simulink model "sunVector_test"  (R2018b)
settings: Solver=VariableStepAuto  StartTime=0.0  StopTime=600  RelTol=1e-3
values from neighbouring files (symbols this model uses):
  utc_test = 137803367    [solarPressure_fullOrbit_test_init.m]    (also in solarPressure_test2_init.m; solarPressure_test_init.m; sunVector_test_init.m = 197208000)
libraries: sunVector_lib x1, time_Lib x1
settings Model: Creator=devantormey  LastModifiedBy=devantormey

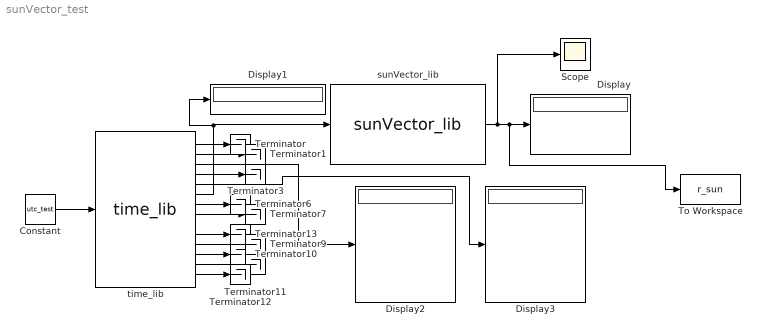
== system sunVector_test ==
  Constant : Constant  Value=utc_test
  Display{,1..3} (4 alike) : Display
  Scope : Scope
  Terminator{,1,3,6..7,9..13} (10 alike) : Terminator
  To Workspace : ToWorkspace  VariableName=r_sun  SaveFormat=Timeseries  SampleTime=-1
  sunVector_lib : sunVector_lib/sunVector_lib  SystemSampleTime=-1
  "time_lib " : time_Lib/time_lib    SystemSampleTime=-1
  wires:
  "time_lib "/3 -> Display2/1
  "time_lib "/12 -> Terminator10/1
  "time_lib "/2 -> Terminator1/1
  "time_lib "/4 -> Terminator3/1
  "time_lib "/13 -> Terminator11/1
  "time_lib "/11 -> Terminator9/1
  "time_lib "/7 -> Terminator6/1
  "time_lib "/8 -> Terminator7/1
  "time_lib "/1 -> Terminator/1
  "time_lib "/14 -> Terminator12/1
  "time_lib "/10 -> Terminator13/1
  Constant/1 -> "time_lib "/1
  "time_lib "/5 -> Display3/1
  "time_lib "/6 -> Display1/1, sunVector_lib/1
  sunVector_lib/1 -> Scope/1, To Workspace/1, Display/1
